simulink model "simulink_neuralEncodingTest"  (R2015a)
settings: Solver=ode45  StartTime=0.0  StopTime=10.0  RelTol=1e-3
undefined symbols (not defined in the file or in its folder): tSamp
libraries: simulink x1
settings Model: Creator=Thomas  LastModifiedBy=Thomas
settings DataIOCC: ExternalInput=tIn  LoadExternalInput=on

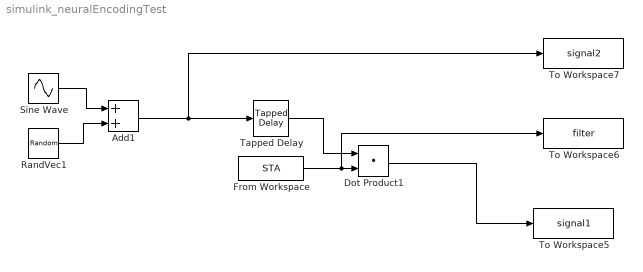
== system simulink_neuralEncodingTest ==
  Add1 : Sum
  Dot Product1 : DotProduct  InputSameDT=on  OutDataTypeStr=Inherit: Inherit via internal rule
  From Workspace : FromWorkspace  VariableName=STA  SampleTime=tSamp
  RandVec1 : RandomNumber  Variance=0.1  SampleTime=tSamp
  Sine Wave : Sin  Frequency=6  SampleTime=tSamp
  Tapped Delay : simulink/Discrete/Tapped Delay  vinit=0.0  samptime=-1  NumDelays=40  DelayOrder=Oldest  includeCurrent=off
  To Workspace5 : ToWorkspace  VariableName=signal1  SaveFormat=Structure With Time  SampleTime=-1
  To Workspace6 : ToWorkspace  VariableName=filter  SaveFormat=Structure With Time  SampleTime=-1
  To Workspace7 : ToWorkspace  VariableName=signal2  SaveFormat=Structure With Time  SampleTime=-1
  wires:
  Sine Wave/1 -> Add1/1
  RandVec1/1 -> Add1/2
  Add1/1 -> To Workspace7/1, Tapped Delay/1
  Tapped Delay/1 -> Dot Product1/1
  From Workspace/1 -> To Workspace6/1, Dot Product1/2
  Dot Product1/1 -> To Workspace5/1
